simulink library "pixhawk_slib_adv"  (R2017b)
settings: Solver=ode45  StartTime=0.0  StopTime=10.0  RelTol=1e-3
undefined symbols (not defined in the file or in its folder): Earth, earthRadius, ModelInit_AngEuler, ModelInit_PosE, ModelInit_RateB, ModelInit_RPM, ModelInit_VelB, ModelParam_envAltitude, ModelParam_GPSLatLong, ModelParam_motorCr, ModelParam_motorJm, ModelParam_motorT, ModelParam_motorWb, ModelParam_noisePowerIMU, ModelParam_rotorCm, ModelParam_rotorCt, ModelParam_uavCCm, ModelParam_uavCd, ModelParam_uavDearo, ModelParam_uavJ, ModelParam_uavMass, ModelParam_uavR, ModelParam_uavType, Receive, Send, WGS84
libraries: etargetslib x11, dspnetwork x9, simulink x8, sharedtransform x5, aerolibtransform2 x4, aerolibutil x4, pixhawk_slib_adv x3, aerolibfltsims x3, shared6dof x1, aerolibobsolete x1, aerolibasang x1, aerolibatmos2 x1
(part 2 of 3)

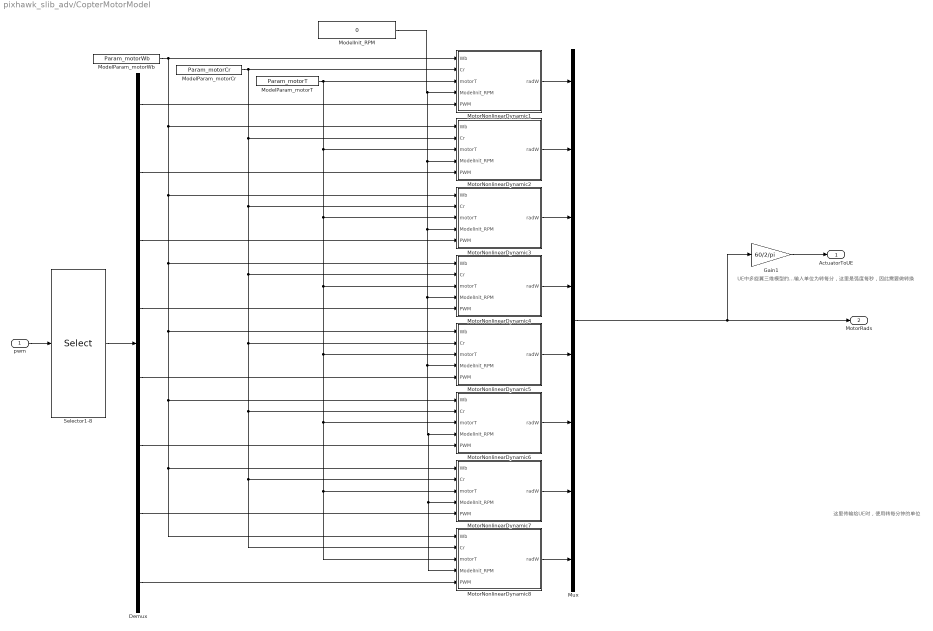
== system pixhawk_slib_adv/CopterMotorModel ==
  note: UE中多旋翼三维模型的输入单位为转每分，这里是弧度每秒，因此需要做转换
  note: 这里传输给UE时，使用转每分钟的单位
  pwm : Inport
  Demux : Demux  Outputs=8
  Gain1 : Gain  Gain=60/2/pi
  ModelInit_RPM : Constant  Value=0
  ModelParam_motorCr : Constant  Value=Param_motorCr
  ModelParam_motorT : Constant  Value=Param_motorT
  ModelParam_motorWb : Constant  Value=Param_motorWb
  MotorNonlinearDynamic1 : Subsystem  TreatAsAtomicUnit=on
  MotorNonlinearDynamic2 : Subsystem  TreatAsAtomicUnit=on
  MotorNonlinearDynamic3 : Subsystem  TreatAsAtomicUnit=on
  MotorNonlinearDynamic4 : Subsystem  TreatAsAtomicUnit=on
  MotorNonlinearDynamic5 : Subsystem  TreatAsAtomicUnit=on
  MotorNonlinearDynamic6 : Subsystem  TreatAsAtomicUnit=on
  MotorNonlinearDynamic7 : Subsystem  TreatAsAtomicUnit=on
  MotorNonlinearDynamic8 : Subsystem  TreatAsAtomicUnit=on
  Mux : Mux  Inputs=8
  Selector1-8 : Selector  InputPortWidth=16  IndexOptions=Index vector (dialog)  Indices=[1:8]  OutputSizes=1
  ActuatorToUE : Outport
  MotorRads : Outport  Port=2
  wires:
  Mux/1 -> Gain1/1, MotorRads/1
  Demux/1 -> MotorNonlinearDynamic1/5(PWM)
  MotorNonlinearDynamic1/1(radW) -> Mux/1
  ModelParam_motorCr/1 -> MotorNonlinearDynamic1/2(Cr), MotorNonlinearDynamic2/2(Cr), MotorNonlinearDynamic3/2(Cr), MotorNonlinearDynamic4/2(Cr), MotorNonlinearDynamic5/2(Cr), MotorNonlinearDynamic6/2(Cr), MotorNonlinearDynamic8/2(Cr), MotorNonlinearDynamic7/2(Cr)
  ModelParam_motorWb/1 -> MotorNonlinearDynamic1/1(Wb), MotorNonlinearDynamic2/1(Wb), MotorNonlinearDynamic3/1(Wb), MotorNonlinearDynamic4/1(Wb), MotorNonlinearDynamic5/1(Wb), MotorNonlinearDynamic6/1(Wb), MotorNonlinearDynamic8/1(Wb), MotorNonlinearDynamic7/1(Wb)
  Demux/2 -> MotorNonlinearDynamic2/5(PWM)
  Demux/3 -> MotorNonlinearDynamic3/5(PWM)
  Demux/4 -> MotorNonlinearDynamic4/5(PWM)
  Demux/5 -> MotorNonlinearDynamic5/5(PWM)
  Demux/6 -> MotorNonlinearDynamic6/5(PWM)
  Demux/7 -> MotorNonlinearDynamic7/5(PWM)
  Demux/8 -> MotorNonlinearDynamic8/5(PWM)
  ModelParam_motorT/1 -> MotorNonlinearDynamic2/3(motorT), MotorNonlinearDynamic3/3(motorT), MotorNonlinearDynamic4/3(motorT), MotorNonlinearDynamic5/3(motorT), MotorNonlinearDynamic6/3(motorT), MotorNonlinearDynamic8/3(motorT), MotorNonlinearDynamic7/3(motorT), MotorNonlinearDynamic1/3(motorT)
  MotorNonlinearDynamic2/1(radW) -> Mux/2
  MotorNonlinearDynamic8/1(radW) -> Mux/8
  MotorNonlinearDynamic7/1(radW) -> Mux/7
  MotorNonlinearDynamic6/1(radW) -> Mux/6
  MotorNonlinearDynamic5/1(radW) -> Mux/5
  MotorNonlinearDynamic4/1(radW) -> Mux/4
  MotorNonlinearDynamic3/1(radW) -> Mux/3
  Selector1-8/1 -> Demux/1
  ModelInit_RPM/1 -> MotorNonlinearDynamic8/4(ModelInit_RPM), MotorNonlinearDynamic7/4(ModelInit_RPM), MotorNonlinearDynamic6/4(ModelInit_RPM), MotorNonlinearDynamic5/4(ModelInit_RPM), MotorNonlinearDynamic4/4(ModelInit_RPM), MotorNonlinearDynamic3/4(ModelInit_RPM), MotorNonlinearDynamic2/4(ModelInit_RPM), MotorNonlinearDynamic1/4(ModelInit_RPM)
  Gain1/1 -> ActuatorToUE/1
  pwm/1 -> Selector1-8/1

== system pixhawk_slib_adv/GroundModel ==
  tz : Inport
  6DOF : Inport  Port=2
  Bus Creator : BusCreator  Inputs=2
  Constant : Constant  Value=ModelChoice
  Multiport Switch : MultiPortSwitch  Inputs=2  DataPortIndices=1
  Subsystem1 : Subsystem
  "Subsystem2 " : Subsystem
  fm : Outport
  wires:
  tz/1 -> Bus Creator/1
  6DOF/1 -> Bus Creator/2
  Multiport Switch/1 -> fm/1
  Constant/1 -> Multiport Switch/1
  Subsystem1/1(Out1) -> Multiport Switch/2
  "Subsystem2 "/1(Out1) -> Multiport Switch/3
  Bus Creator/1 -> "Subsystem2 "/1(In1), Subsystem1/1(In1)

== system pixhawk_slib_adv/PX4FaultInParamsSend ==
  note: struct PX4ModelInParams {
      | int checksum ; //1234567891
      | int Bitmask ;
      | double InParams [ 32 ];
      | };
  note: This message will be sent to PX4 DLL model's Params signals ModelInParams [32].
      | The checksum should be set to 1234567891, and the data should be sent to port 30100+(i-1)*2.
      | The bitmask specify which dimension of 32-D ModelInParams vector.
  Bitmask : Inport  OutDataTypeStr=int32  PortDimensions=1
  InParams : Inport  Port=2  OutDataTypeStr=single  PortDimensions=32
  Data Type Conversion1 : DataTypeConversion  OutDataTypeStr=int32
  Data Type Conversion2 : DataTypeConversion  OutDataTypeStr=double
  Data Type Conversion3 : DataTypeConversion  OutDataTypeStr=int32
  PayLoad : etargetslib/Byte Pack  datatypes={'int32','int32','double'}  byteAlign=4
  UDP Send : dspnetwork/UDP Send  remoteURL=TargetIP  remotePort=30100 + CopterID*2 -2  localURL='0.0.0.0'  localPortSource=Automatically determine  localPort=-1  sampletime=-1  blockPlatform=[]  separateLengthPort=0
      settings: SourceProductName=DSP System Toolbox  SourceProductBaseCode=DS
  checksum : Constant  Value=1234567891  OutDataTypeStr=Inherit: Inherit via back propagation
  wires:
  InParams/1 -> Data Type Conversion2/1
  Bitmask/1 -> Data Type Conversion1/1
  PayLoad/1 -> UDP Send/1
  Data Type Conversion1/1 -> PayLoad/2
  Data Type Conversion2/1 -> PayLoad/3
  checksum/1 -> Data Type Conversion3/1
  Data Type Conversion3/1 -> PayLoad/1

== system pixhawk_slib_adv/PX4SILIntFloatSend ==
  note: struct PX4SILIntFloat {
      | int checksum ;
      | int CopterID ;
      | int inSILInts [ 8 ];
      | float inSILFLoats [ 20 ];
      | }
  note: This message will be sent to PX4 DLL model's input signals inSILInts[8] and inSILFloats[20].
      | The checksum should be set to 1234567897, and the data should be sent to port 30100+(i-1)*2
  inSILInts : Inport  OutDataTypeStr=int32  PortDimensions=8
  inSILFloats : Inport  Port=2  OutDataTypeStr=single  PortDimensions=20
  CopterID : Constant  OutDataTypeStr=Inherit: Inherit via back propagation
  Data Type Conversion1 : DataTypeConversion  OutDataTypeStr=int32
  Data Type Conversion2 : DataTypeConversion  OutDataTypeStr=single
  Data Type Conversion3 : DataTypeConversion  OutDataTypeStr=int32
  Mux : Mux  Inputs=2
  PayLoad : etargetslib/Byte Pack  datatypes={'int32','int32','single'}  byteAlign=8
  UDP Send : dspnetwork/UDP Send  remoteURL=TargetIP  remotePort=30100 + CopterID*2 -2  localURL='0.0.0.0'  localPortSource=Automatically determine  localPort=-1  sampletime=-1  blockPlatform=[]  separateLengthPort=0
      settings: SourceProductName=DSP System Toolbox  SourceProductBaseCode=DS
  checksum : Constant  Value=1234567897  OutDataTypeStr=Inherit: Inherit via back propagation
  wires:
  inSILFloats/1 -> Data Type Conversion2/1
  inSILInts/1 -> Data Type Conversion1/1
  PayLoad/1 -> UDP Send/1
  Data Type Conversion1/1 -> PayLoad/2
  Data Type Conversion2/1 -> PayLoad/3
  checksum/1 -> Mux/1
  Mux/1 -> Data Type Conversion3/1
  Data Type Conversion3/1 -> PayLoad/1
  CopterID/1 -> Mux/2

== system pixhawk_slib_adv/PlaneGroundModel ==
  note: GroundSupportModel
  note: From Earth to body frame
  note: 计算重量
  "tZ " : Inport
  6DOF : Inport  Port=2
  Bus Selector : BusSelector  OutputSignals=Xe,Ve,Eular(rad),DCM,wb,mass,gravity
  Direction Cosine Matrix to Quaternions : sharedtransform/Direction Cosine Matrix  to Quaternions
      settings: SourceProductName=Aerospace Blockset  SourceProductBaseCode=AE
  Direction Cosine Matrix to Quaternions1 : sharedtransform/Direction Cosine Matrix  to Quaternions
      settings: SourceProductName=Aerospace Blockset  SourceProductBaseCode=AE
  Euler to DCM : aerolibtransform2/Wind Angles to  Direction Cosine Matrix
      settings: SourceProductName=Aerospace Blockset  SourceProductBaseCode=AE
  Ground Model : MATLAB Function  TreatAsAtomicUnit=on
  Mux : Mux  Inputs=2
  OnGroundFaceup : Subsystem
  Product : Product  Multiplication=Matrix(*)
  Product1 : Product
  Quaternion Inverse : aerolibutil/Quaternion Inverse
      settings: SourceProductName=Aerospace Blockset
  Quaternion Multiplication : aerolibutil/Quaternion Multiplication
  FM : Outport
  wires:
  "tZ "/1 -> Ground Model/6(terrainZ)
  Ground Model/2(M1) -> Mux/2  "Mb"
  Product/1 -> Mux/1  "Fb"
  Quaternion Multiplication/1 -> Ground Model/5(Quet)
  Quaternion Inverse/1 -> Quaternion Multiplication/1
  Direction Cosine Matrix to Quaternions1/1 -> Quaternion Inverse/1
  Euler to DCM/1 -> Direction Cosine Matrix to Quaternions1/1
  Direction Cosine Matrix to Quaternions/1 -> Quaternion Multiplication/2
  Ground Model/1(F1) -> Product/2
  Bus Selector/4 -> Direction Cosine Matrix to Quaternions/1, Product/1  "<DCM>"
  Bus Selector/5 -> Ground Model/2(wb)  "<wb>"
  6DOF/1 -> Bus Selector/1
  Bus Selector/2 -> Ground Model/4(Ve)  "<Ve>"
  Bus Selector/1 -> Ground Model/3(Xe)  "<Xe>"
  Bus Selector/3 -> OnGroundFaceup/1(Eular(rad))  "<Eular(rad)>"
  OnGroundFaceup/1(y) -> Euler to DCM/1
  Product1/1 -> Ground Model/1(mg)  "mg"
  Bus Selector/6 -> Product1/1  "<mass>"
  Bus Selector/7 -> Product1/2  "<gravity>"
  Mux/1 -> FM/1

== system pixhawk_slib_adv/RflyChangeMap ==
  MapNameorID : Inport
  Data Type Conversion8 : DataTypeConversion  OutDataTypeStr=int32
  Data Type Conversion9 : DataTypeConversion  OutDataTypeStr=uint8
  MATLAB Function : MATLAB Function  TreatAsAtomicUnit=on
  PayLoad1 : etargetslib/Byte Pack  datatypes={'int32','uint8'}  byteAlign=4
  UDP Send1 : dspnetwork/UDP Send  remoteURL='127.0.0.1'  remotePort=20010  localURL='0.0.0.0'  localPortSource=Automatically determine  localPort=-1  sampletime=-1  blockPlatform=[]  separateLengthPort=0
      settings: SourceProductName=DSP System Toolbox  SourceProductBaseCode=DS
  checkSum : Constant  Value=1234567890
  wires:
  MapNameorID/1 -> MATLAB Function/1(input)
  checkSum/1 -> Data Type Conversion8/1
  Data Type Conversion9/1 -> PayLoad1/2
  PayLoad1/1 -> UDP Send1/1
  Data Type Conversion8/1 -> PayLoad1/1
  MATLAB Function/1(data) -> Data Type Conversion9/1

== system pixhawk_slib_adv/SensorOutput ==
  note: Struct MavHILStateQuat{
      | uint64_t time_usec; /*< Timestamp (microseconds since UNIX epoch or microseconds since system boot)*/
      | float attitude_quaternion [ 4 ]; /*< Vehicle attitude expressed as normalized quaternion in w, x, y, z order (with 1 0 0 0 being the null-rotation)*/
      | float rollspeed; /*< Body frame roll / phi angular speed (rad/s)*/
      | float pitchspeed; /*< Body frame pitch / theta angular speed (rad/s)*/
      | float yawspeed; /*< Body frame yaw / psi angular speed (rad/s)*/
      | int32_t lat; /*< Latitude, expressed as * 1E7*/
      | int32_t lon; /*< Longitude, expressed as * 1E7*/
      | int32_t alt; /*< Altitude in meters, expressed as * 1000 (millimeters)*/
      | int16_t vx; /*< Ground X Speed (Latitude), expressed as cm/s*/
      | int16_t vy; /*< Ground Y Speed (Longitude), expressed as cm/s*/
      | int16_t vz; /*< Ground Z Speed (Altitude), expressed as cm/s*/
      | uint16_t ind_airspeed; /*< Indicated airspeed, expressed as cm/s*/
      | uint16_t true_airspeed; /*< True airspeed, expressed as cm/s*/
      | int16_t xacc; /*< X acceleration (mg)*/
      | int16_t yacc; /*< Y acceleration (mg)*/
      | int16_t zacc; /*< Z acceleration (mg)*/
      | };
  6DOF : Inport
  Bus Selector : BusSelector  OutputSignals=Ve,DCM,wb,dwb/dt,AccB,WindB,PosGPS,gravity
  Clock1 : Clock
  Gain_clock : Gain  Gain=1E6
  HILGPSModel : Subsystem
  HILSensorMavModel : Subsystem
  HILSensor30d : Outport
  HILGPS30d : Outport  Port=2
  wires:
  Bus Selector/8 -> HILSensorMavModel/2(Gravity)  "<gravity>"
  Bus Selector/2 -> HILSensorMavModel/7(DCMbe)  "<DCM>"
  Bus Selector/4 -> HILSensorMavModel/5(dwt)  "<dwb/dt>"
  Bus Selector/7 -> HILSensorMavModel/3(GPSPos), HILGPSModel/3(PosGPS)  "<PosGPS>"
  Bus Selector/5 -> HILSensorMavModel/6(Ab)  "<AccB>"
  Bus Selector/1 -> HILGPSModel/2(Ve)  "<Ve>"
  Bus Selector/3 -> HILSensorMavModel/4(wb)  "<wb>"
  6DOF/1 -> Bus Selector/1
  Clock1/1 -> Gain_clock/1
  Gain_clock/1 -> HILSensorMavModel/1(time_usec), HILGPSModel/1(time_usec)  "time_usec"
  Bus Selector/6 -> HILSensorMavModel/8(windB)  "<WindB>"
  HILSensorMavModel/1(HILSensor30d) -> HILSensor30d/1
  HILGPSModel/1(HILGPS30d) -> HILGPS30d/1

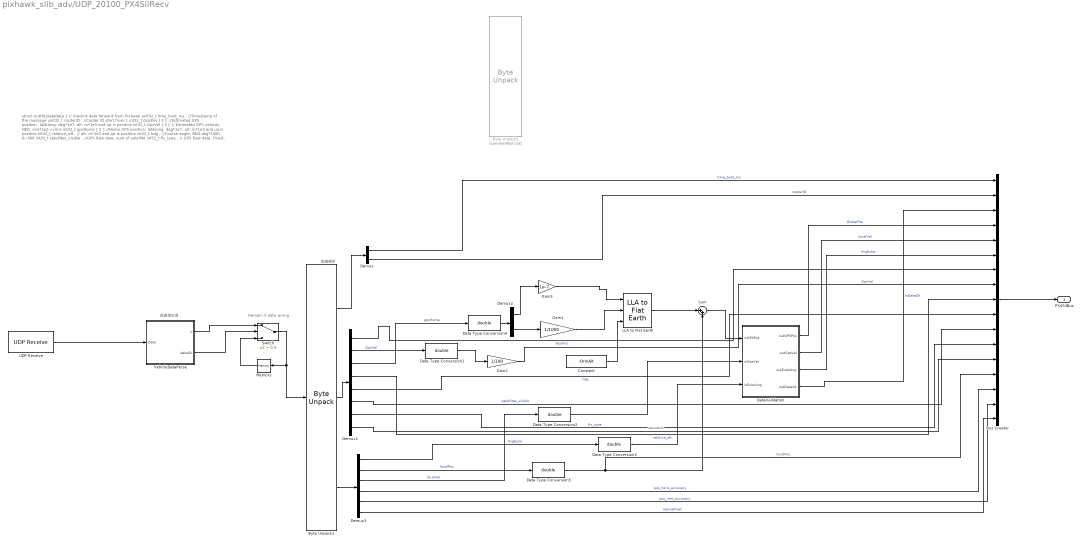
== system pixhawk_slib_adv/UDP_20100_PX4SilRecv ==
  note: 数据解析
  note: 数据预处理
  note: Remain if data wrong
  note: struct outHILStateData { // mavlink data forward from Pixhawk
      | uint32_t time_boot_ms ; //Timestamp of the message
      | uint32_t copterID ; //Copter ID start from 1
      | int32_t GpsPos [ 3 ]; //Estimated GPS position，lat&long: deg*1e7, alt: m*1e3 and up is positive
      | int32_t GpsVel [ 3 ]; // Estimated GPS velocity, NED, m/s*1e2->cm/s
      | int32_t gpsHome [ 3 ]; //Home GPS position, lat&long: deg*1e7, alt: m*1e3 and up is positive
      | int32_t relative_alt ; // alt: m*1e3 and up is positive
      | int32_t hdg ; //Course angle, NED,deg*1000, 0~360
      | int32_t satellites_visible ; //GPS Raw data, sum of satellite
      | int32_t fix_type ; // GPS Raw data, Fixed type, 3 for fixed (good precision)
      | int32_t resrveInit ; //Int, reserve for the future use
      | float AngEular [ 3 ]; //Estimated Euler angle, unit: rad/s
      | float localPos [ 3 ]; //Estimated locoal position, NED, unit: m
      | float localVel [ 3 ]; // Estimated locoal velocity, NED, unit: m/s
      | float pos_horiz_accuracy ; // GPS horizontal accuracy, unit: m
      | float pos_vert_accuracy ; // GPS vertical accuracy, unit: m
      | float resrveFloat ; //float, reserve for the future use
      | }
  Bus Creator : BusCreator  Inputs=17
  Byte Unpack1 : etargetslib/Byte Unpack  dimensions={2,14,12}  datatypes={'uint32','int32','single'}  byteAlign=8
  Byte Unpack2 : etargetslib/Byte Unpack  Commented=on  dimensions={1,1,1,3,3,3,4,8,3,3,3}  datatypes={'int32','int32','double','single','single','single','single','single','single','single','double'}  byteAlign=1
  Constant : Constant  Value=-OrinAlt
  Data Type Conversion{1..5} (5 alike) : DataTypeConversion  OutDataTypeStr=double
  DataValidation : MATLAB Function  TreatAsAtomicUnit=on
  Demux : Demux  Outputs=2
  Demux1 : Demux  Outputs=[3,3,3,1,1,1,1,1]
  Demux2 : Demux  Outputs=[2,1]
  Demux3 : Demux  Outputs=[3,3,3,1,1,1]
  Gain1 : Gain  Gain=1/1000
  Gain2 : Gain  Gain=1/100
  Gain5 : Gain  Gain=1e-7
  LLA to Flat Earth : aerolibtransform2/LLA to Flat Earth  units=Metric (MKS)  ptype=Earth (WGS84)  F=1/298.257223563  R=6378137  LL0=OrinLatLon  psi=0
      settings: SourceProductName=Aerospace Blockset  SourceProductBaseCode=AE
  Memory : Memory  InitialCondition=uint8(zeros(112,1))
  Sum : Sum  Inputs=|++
  Switch : Switch  Criteria=u2 > Threshold  Threshold=0.5
  UDP Receive : dspnetwork/UDP Receive  localURL='0.0.0.0'  localPort=20100 + CopterID*2 -1  remoteURL='0.0.0.0'  remotePort=-1  recvBufferSize=8192  dims=255  signalDatatype=uint8  isVarSize=on  showBlockingTime=off  blockingTime=0  sampletime=-1  blockPlatform=[]
      settings: SourceProductName=DSP System Toolbox  SourceProductBaseCode=DS
  VehicleDataPerse : MATLAB Function  TreatAsAtomicUnit=on
  PX4SilBus : Outport
  wires:
  VehicleDataPerse/2(dataOk) -> Switch/2
  UDP Receive/1 -> VehicleDataPerse/1(Data)
  VehicleDataPerse/1(y) -> Switch/1
  Switch/1 -> Memory/1, Byte Unpack1/1
  Memory/1 -> Switch/3
  Byte Unpack1/1 -> Demux/1
  Demux/1 -> Bus Creator/1  "time_boot_ms"
  Demux/2 -> Bus Creator/2  "copterID"
  Byte Unpack1/2 -> Demux1/1
  Demux1/2 -> Data Type Conversion1/1  "GpsVel"
  Demux2/1 -> Gain5/1
  Demux2/2 -> Gain1/1
  Gain1/1 -> LLA to Flat Earth/2
  Demux1/1 -> Bus Creator/7  "GpsPos"
  LLA to Flat Earth/1 -> Sum/1
  Data Type Conversion1/1 -> Gain2/1
  Data Type Conversion3/1 -> DataValidation/3(inEulerAng)
  Gain5/1 -> LLA to Flat Earth/1
  Data Type Conversion4/1 -> Demux2/1
  Byte Unpack1/3 -> Demux3/1
  Demux1/3 -> Data Type Conversion4/1  "gpsHome"
  Demux1/4 -> Bus Creator/9  "relative_alt"
  Demux1/5 -> Bus Creator/10  "hdg"
  Demux1/6 -> Bus Creator/11  "satellites_visible"
  Demux1/7 -> Bus Creator/12  "fix_type"
  Demux3/1 -> Data Type Conversion3/1  "AngEular"
  Demux3/2 -> Data Type Conversion5/1  "localPos"
  Demux3/3 -> Data Type Conversion2/1  "localVel"
  Demux3/4 -> Bus Creator/15  "pos_horiz_accuracy"
  Demux3/5 -> Bus Creator/16  "pos_vert_accuracy"
  Demux1/8 -> Bus Creator/13  "resrveInit"
  Demux3/6 -> Bus Creator/17  "resrveFloat"
  Constant/1 -> LLA to Flat Earth/3
  DataValidation/1(outGPSPos) -> Bus Creator/4  "GlobalPos"
  DataValidation/2(outGpsVel) -> Bus Creator/5  "localVel"
  DataValidation/3(outEulerAng) -> Bus Creator/6  "AngEular"
  DataValidation/4(outDataOk) -> Bus Creator/3  "IsDataOK"
  Data Type Conversion2/1 -> DataValidation/2(inGpsVel)
  Gain2/1 -> Bus Creator/8  "GpsVel"
  Data Type Conversion5/1 -> Bus Creator/14, Sum/2  "localPos"
  Sum/1 -> DataValidation/1(inGPSPos)
  Bus Creator/1 -> PX4SilBus/1

== system pixhawk_slib_adv/UDP_30100_TrueSimRecv ==
  note: % //FULL完整模式，输出到RflySim3D的数据
      | % struct SOut2Simulator {
      | %     int checksum; // 校验码123456789，必须设定为本值，才会认为是有效数据
      | %     int copterID;  //飞机ID序号
      | %     int vehicleType;  //载具样式ID，对应UE的XML中ClassID
      | %     int reserv; //备用标志位，Int型，将来用于表示碰撞、或大地图等标识
      | %     float VelE[3];   //速度，北东地，单位米/s
      | %     float AngEuler[3];  //欧拉角，滚转俯仰偏航，单位弧度
      | %     float AngQuatern[4]; //姿态四元数向量，w x y z
      | %     float MotorRPMS[8];  //执行器偏转量或转速，旋翼类对应RPM转每分
      | %     float AccB[3];       //载具机体FRD坐标系下加速度
      | %     float RateB[3];      //载具机体FRD坐标系下角速度，pqr，单位rad/s
      | %     double runnedTime; //时间戳，仿真开始为0时刻。
      | %     double PosE[3];   //北东地位置，单位米，z向下为正
      | %     double PosGPS[3];    //载具纬度、经度、高度向量，单位度和米，高度向上为正
      | % };
      | % // Python解码标识4i24f7d，数据长度168字节
  note: 数据解析
  Bus Creator : BusCreator  Inputs=13
  Demux2 : Demux  Outputs=35
  Mux{,1,4..7} (6 alike) : Mux  Inputs=3
  Mux2 : Mux
  Mux3 : Mux  Inputs=8
  Terminator : Terminator
  UDP Receive : dspnetwork/UDP Receive  localURL='0.0.0.0'  localPort=30100 + CopterID * 2 -1  remoteURL='0.0.0.0'  remotePort=-1  recvBufferSize=8192  dims=255  signalDatatype=uint8  isVarSize=on  showBlockingTime=off  blockingTime=0  sampletime=-1  blockPlatform=[]
      settings: SourceProductName=DSP System Toolbox  SourceProductBaseCode=DS
  VehicleDataPerse1 : MATLAB Function  TreatAsAtomicUnit=on
  SimData : Outport
  wires:
  UDP Receive/1 -> VehicleDataPerse1/1(Data)
  VehicleDataPerse1/1(y) -> Demux2/1
  Demux2/2 -> Bus Creator/1  "copterID"
  Demux2/3 -> Bus Creator/2  "vehicleType"
  Demux2/4 -> Bus Creator/3  "reserv"
  Demux2/5 -> Mux/1
  Demux2/6 -> Mux/2
  Demux2/7 -> Mux/3
  Mux/1 -> Bus Creator/4  "VelE"
  Demux2/8 -> Mux1/1
  Demux2/9 -> Mux1/2
  Demux2/10 -> Mux1/3
  Mux1/1 -> Bus Creator/5  "AngEuler"
  Demux2/11 -> Mux2/1
  Demux2/12 -> Mux2/2
  Demux2/13 -> Mux2/3
  Demux2/14 -> Mux2/4
  Mux2/1 -> Bus Creator/6  "AngQuatern"
  Demux2/15 -> Mux3/1
  Demux2/16 -> Mux3/2
  Demux2/17 -> Mux3/3
  Demux2/18 -> Mux3/4
  Demux2/19 -> Mux3/5
  Demux2/20 -> Mux3/6
  Demux2/21 -> Mux3/7
  Demux2/22 -> Mux3/8
  Mux3/1 -> Bus Creator/7  "MotorRPMS"
  Demux2/23 -> Mux4/1
  Demux2/24 -> Mux4/2
  Demux2/25 -> Mux4/3
  Mux4/1 -> Bus Creator/8  "AccB"
  Demux2/26 -> Mux5/1
  Demux2/27 -> Mux5/2
  Demux2/28 -> Mux5/3
  Mux5/1 -> Bus Creator/9  "RateB"
  Demux2/29 -> Bus Creator/10  "runnedTime"
  Demux2/30 -> Mux6/1
  Demux2/31 -> Mux6/2
  Demux2/32 -> Mux6/3
  Mux6/1 -> Bus Creator/11  "PosE"
  Demux2/33 -> Mux7/1
  Demux2/34 -> Mux7/2
  Demux2/35 -> Mux7/3
  Mux7/1 -> Bus Creator/12  "PosGPS"
  Bus Creator/1 -> SimData/1
  Demux2/1 -> Terminator/1
  VehicleDataPerse1/2(dataOk) -> Bus Creator/13  "IsDataOK"

== system pixhawk_slib_adv/UDP_40100_RflyPx4Recv ==
  note: struct PX4ExtMsg {
      | int checksum ; //1234567898
      | int CopterID ;
      | double runnedTime ; //Current stamp (s)
      | float controls [ 8 ];
      | }
  note: 数据解析
  note: 数据预处理
  note: 如果数据不正确则用前一时刻数据
  Byte Unpack1 : etargetslib/Byte Unpack  dimensions={2,1,8}  datatypes={'int32','double','single'}  byteAlign=8
  CopterID : Display
  Demux : Demux  Outputs=2
  Memory : Memory  InitialCondition=uint8(zeros(48,1))
  Switch : Switch  Criteria=u2 > Threshold  Threshold=0.5
  UDP Receive : dspnetwork/UDP Receive  localURL='0.0.0.0'  localPort=40100 + CopterID * 2 -1  remoteURL='0.0.0.0'  remotePort=-1  recvBufferSize=8192  dims=120  signalDatatype=uint8  isVarSize=on  showBlockingTime=off  blockingTime=0  sampletime=-1  blockPlatform=[]
      settings: SourceProductName=DSP System Toolbox  SourceProductBaseCode=DS
  VehicleDataPerse : MATLAB Function  TreatAsAtomicUnit=on
  checksum : Display
  runnedTime : Display
  controls : Outport
  wires:
  VehicleDataPerse/2(dataOk) -> Switch/2
  UDP Receive/1 -> VehicleDataPerse/1(Data)
  VehicleDataPerse/1(y) -> Switch/1
  Switch/1 -> Memory/1, Byte Unpack1/1
  Memory/1 -> Switch/3
  Byte Unpack1/1 -> Demux/1
  Demux/1 -> checksum/1
  Demux/2 -> CopterID/1
  Byte Unpack1/2 -> runnedTime/1
  Byte Unpack1/3 -> controls/1

== system pixhawk_slib_adv/sendUE4ExtAct ==
  CopterID : Inport
  "ActExt  " : Inport  Port=2
  UDP Send2 : dspnetwork/UDP Send  remoteURL='127.0.0.1'  remotePort=20010  localURL='0.0.0.0'  localPortSource=Automatically determine  localPort=-1  sampletime=-1  blockPlatform=[]  separateLengthPort=0
      settings: SourceProductName=DSP System Toolbox  SourceProductBaseCode=DS
  Ue4ExtMsgEncoder : Subsystem
  wires:
  CopterID/1 -> Ue4ExtMsgEncoder/1(copterID)
  "ActExt  "/1 -> Ue4ExtMsgEncoder/2(pwm)
  Ue4ExtMsgEncoder/1(Ue4ExtMsg) -> UDP Send2/1

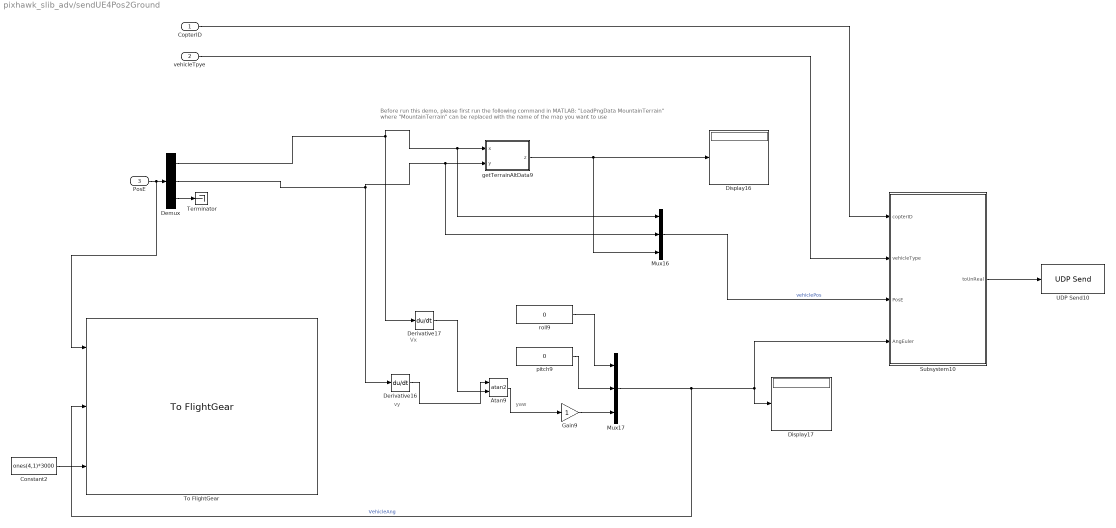
== system pixhawk_slib_adv/sendUE4Pos2Ground ==
  note: vy
  note: Vx
  note: Before run this demo, please first run the following command in MATLAB: "LoadPngData MountainTerrain"
      | where "MountainTerrain" can be replaced with the name of the map you want to use
  note: yaw
  CopterID : Inport
  vehicleTpye : Inport  Port=2
  PosE : Inport  Port=3
  Atan9 : Trigonometry  Operator=atan2
  Constant2 : Constant  Value=ones(4,1)*3000
  Demux : Demux  Outputs=3
  Derivative16 : Derivative
  Derivative17 : Derivative
  Display16 : Display
  Display17 : Display
  Gain9 : Gain
  Mux16 : Mux  Inputs=3
  Mux17 : Mux  Inputs=3
  Subsystem10 : Subsystem
  Terminator : Terminator
  To FlightGear : pixhawk_slib_adv/sendUE4PosFull/To FlightGear  SystemSampleTime=-1  Latency=0  AutoFrameSizeCalculation=off
      settings: SourceProductName=Pixhawk Target Blocks
  UDP Send10 : dspnetwork/UDP Send  remoteURL='127.0.0.1'  remotePort=20010  localURL='0.0.0.0'  localPortSource=Automatically determine  localPort=-1  sampletime=-1  blockPlatform=[]  separateLengthPort=0
      settings: SourceProductName=DSP System Toolbox  SourceProductBaseCode=DS
  getTerrainAltData9 : MATLAB Function  TreatAsAtomicUnit=on
  pitch9 : Constant  Value=0
  roll9 : Constant  Value=0
  wires:
  pitch9/1 -> Mux17/2
  Gain9/1 -> Mux17/3
  Mux17/1 -> To FlightGear/2, Display17/1, Subsystem10/4(AngEuler)  "VehicleAng"
  Derivative17/1 -> Atan9/2
  Demux/2 -> Derivative16/1, Mux16/2, getTerrainAltData9/2(y)
  vehicleTpye/1 -> Subsystem10/2(vehicleType)
  CopterID/1 -> Subsystem10/1(copterID)
  Subsystem10/1(toUnReal) -> UDP Send10/1
  Atan9/1 -> Gain9/1
  roll9/1 -> Mux17/1
  Demux/1 -> Mux16/1, getTerrainAltData9/1(x), Derivative17/1
  Derivative16/1 -> Atan9/1
  Mux16/1 -> Subsystem10/3(PosE)  "vehiclePos"
  getTerrainAltData9/1(z) -> Mux16/3, Display16/1
  PosE/1 -> To FlightGear/1, Demux/1
  Demux/3 -> Terminator/1
  Constant2/1 -> To FlightGear/3

== system pixhawk_slib_adv/sendUE4PosFull ==
  copterID : Inport  PortDimensions=1
  vehicleType : Inport  Port=2  PortDimensions=1
  MotorRPMS : Inport  Port=3
  VelE : Inport  Port=4
  PosE : Inport  Port=5  PortDimensions=3
  RateB : Inport  Port=6
  AngEuler : Inport  Port=7  PortDimensions=3
  Clock : Clock
  Constant1 : Constant  Value=[0,0,0,0]
  Constant3 : Constant  Value=[0,0,0]
  Constant5 : Constant  Value=[0,0,0]
  Subsystem : Subsystem
  To FlightGear : Subsystem
      mask Display: image('./icon/FlightGear.png');
  UDP Send : dspnetwork/UDP Send  remoteURL='127.0.0.1'  remotePort=20010  localURL='0.0.0.0'  localPortSource=Automatically determine  localPort=-1  sampletime=-1  blockPlatform=[]  separateLengthPort=0
      settings: SourceProductName=DSP System Toolbox  SourceProductBaseCode=DS
  wires:
  RateB/1 -> Subsystem/10(RateB)
  Constant5/1 -> Subsystem/11(PosGPS)
  Constant3/1 -> Subsystem/9(AccB)
  Subsystem/1(toUnReal) -> UDP Send/1
  VelE/1 -> Subsystem/4("VelE ")
  Clock/1 -> Subsystem/3(runnedTime)
  MotorRPMS/1 -> To FlightGear/3(MotorPWMs), Subsystem/8(MotorRPMS)
  Constant1/1 -> Subsystem/7(AngQuatern)
  AngEuler/1 -> To FlightGear/2(AngEuler), Subsystem/6(AngEuler)
  PosE/1 -> To FlightGear/1(PosE), Subsystem/5(PosE)
  copterID/1 -> Subsystem/1(copterID)
  vehicleType/1 -> Subsystem/2(vehicleType)

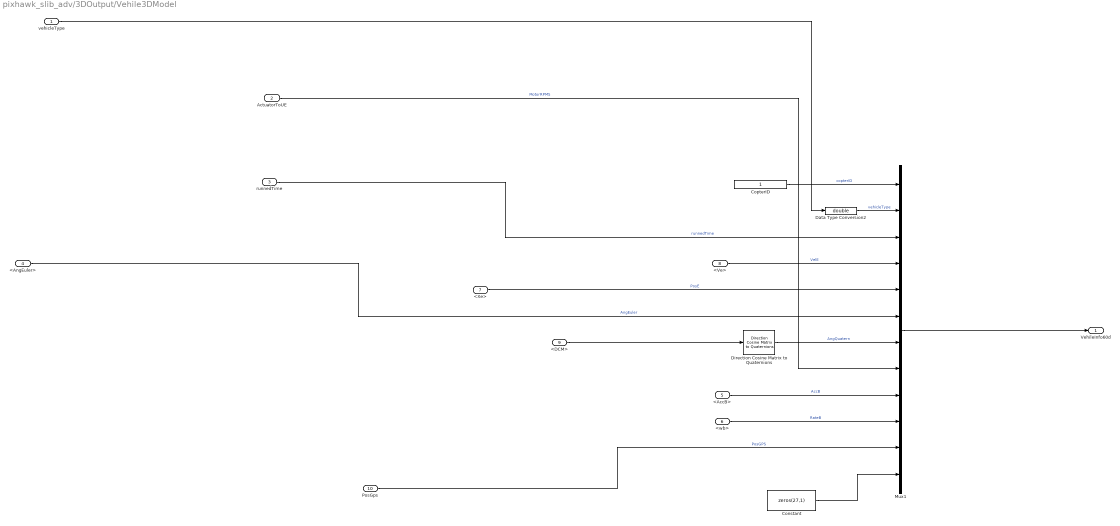
== system pixhawk_slib_adv/3DOutput/Vehile3DModel ==
  vehicleType : Inport
  ActuatorToUE : Inport  Port=2
  runnedTime : Inport  Port=3
  <AngEuler> : Inport  Port=4
  <AccB> : Inport  Port=5
  <wb> : Inport  Port=6
  <Xe> : Inport  Port=7
  <Ve> : Inport  Port=8
  <DCM> : Inport  Port=9
  PosGps : Inport  Port=10
  Constant : Constant  Value=zeros(27,1)
  CopterID : Constant
  Data Type Conversion2 : DataTypeConversion  OutDataTypeStr=double
  Direction Cosine Matrix to Quaternions : sharedtransform/Direction Cosine Matrix  to Quaternions
      settings: SourceProductName=Aerospace Blockset  SourceProductBaseCode=AE
  Mux1 : Mux  Inputs=12
  VehileInfo60d : Outport
  wires:
  Mux1/1 -> VehileInfo60d/1
  Data Type Conversion2/1 -> Mux1/2  "vehicleType"
  runnedTime/1 -> Mux1/3  "runnedTime"
  <AccB>/1 -> Mux1/9  "AccB"
  CopterID/1 -> Mux1/1  "copterID"
  Direction Cosine Matrix to Quaternions/1 -> Mux1/7  "AngQuatern"
  <wb>/1 -> Mux1/10  "RateB"
  <AngEuler>/1 -> Mux1/6  "AngEuler"
  <Xe>/1 -> Mux1/5  "PosE"
  vehicleType/1 -> Data Type Conversion2/1
  <Ve>/1 -> Mux1/4  "VelE"
  ActuatorToUE/1 -> Mux1/8  "MotorRPMS"
  <DCM>/1 -> Direction Cosine Matrix to Quaternions/1
  Constant/1 -> Mux1/12
  PosGps/1 -> Mux1/11  "PosGPS"

== system pixhawk_slib_adv/CopterGroundModel/OnGroundFaceup ==
  Eular(rad) : Inport
  ModelInit_GroundSlope : Constant  Value=[0,0]
  Mux : Mux  Inputs=2
  Selector : Selector  InputPortWidth=3  IndexOptions=Index vector (dialog)  Indices=[3]  OutputSizes=1
  y : Outport
  wires:
  Mux/1 -> y/1
  ModelInit_GroundSlope/1 -> Mux/1
  Selector/1 -> Mux/2
  Eular(rad)/1 -> Selector/1

== system pixhawk_slib_adv/CopterMotorModel/MotorNonlinearDynamic1 ==
  Wb : Inport
  Cr : Inport  Port=2
  motorT : Inport  Port=3
  ModelInit_RPM : Inport  Port=4
  PWM : Inport  Port=5
  Minimum Throttle Cutoff : simulink/Logic and Bit Operations/Compare To Constant  relop=>=  const=ModelParam_motorMinThr  OutDataTypeStr=uint8
  Motor_Dynamics : Subsystem  TreatAsAtomicUnit=on
  Motor_Dynamics_backup : StateSpace  Commented=on  A=-1/ModelParam_motorT  C=1/ModelParam_motorT  D=0  InitialCondition=ModelInit_RPM*ModelParam_motorT
  Product : Product
  Product1 : Product
  Signal_Saturation : Saturate  UpperLimit=0.95  LowerLimit=0
  Sum1 : Sum  Inputs=++|
  radW : Outport
  wires:
  PWM/1 -> Signal_Saturation/1
  Motor_Dynamics/1(motor_rate_act) -> radW/1
  Product/1 -> Motor_Dynamics/1(motor_rate_d)
  Signal_Saturation/1 -> Product1/2, Minimum Throttle Cutoff/1
  Product1/1 -> Sum1/2
  Sum1/1 -> Product/1
  Wb/1 -> Sum1/1
  Minimum Throttle Cutoff/1 -> Product/2
  Cr/1 -> Product1/1
  motorT/1 -> Motor_Dynamics/3(motorT)
  ModelInit_RPM/1 -> Motor_Dynamics/2(ModelInit_RPM)

== system pixhawk_slib_adv/CopterMotorModel/MotorNonlinearDynamic2 ==
  Wb : Inport
  Cr : Inport  Port=2
  motorT : Inport  Port=3
  ModelInit_RPM : Inport  Port=4
  PWM : Inport  Port=5
  Minimum Throttle Cutoff : simulink/Logic and Bit Operations/Compare To Constant  relop=>=  const=ModelParam_motorMinThr  OutDataTypeStr=uint8
  Motor_Dynamics : Subsystem  TreatAsAtomicUnit=on
  Motor_Dynamics_backup : StateSpace  Commented=on  A=-1/ModelParam_motorT  C=1/ModelParam_motorT  D=0  InitialCondition=ModelInit_RPM*ModelParam_motorT
  Product : Product
  Product1 : Product
  Signal_Saturation : Saturate  UpperLimit=0.95  LowerLimit=0
  Sum1 : Sum  Inputs=++|
  radW : Outport
  wires:
  ModelInit_RPM/1 -> Motor_Dynamics/2(ModelInit_RPM)
  motorT/1 -> Motor_Dynamics/3(motorT)
  Cr/1 -> Product1/1
  Minimum Throttle Cutoff/1 -> Product/2
  Wb/1 -> Sum1/1
  Sum1/1 -> Product/1
  Product1/1 -> Sum1/2
  Signal_Saturation/1 -> Minimum Throttle Cutoff/1, Product1/2
  Product/1 -> Motor_Dynamics/1(motor_rate_d)
  Motor_Dynamics/1(motor_rate_act) -> radW/1
  PWM/1 -> Signal_Saturation/1

== system pixhawk_slib_adv/CopterMotorModel/MotorNonlinearDynamic3 ==
  Wb : Inport
  Cr : Inport  Port=2
  motorT : Inport  Port=3
  ModelInit_RPM : Inport  Port=4
  PWM : Inport  Port=5
  Minimum Throttle Cutoff : simulink/Logic and Bit Operations/Compare To Constant  relop=>=  const=ModelParam_motorMinThr  OutDataTypeStr=uint8
  Motor_Dynamics : Subsystem  TreatAsAtomicUnit=on
  Motor_Dynamics_backup : StateSpace  Commented=on  A=-1/ModelParam_motorT  C=1/ModelParam_motorT  D=0  InitialCondition=ModelInit_RPM*ModelParam_motorT
  Product : Product
  Product1 : Product
  Signal_Saturation : Saturate  UpperLimit=0.95  LowerLimit=0
  Sum1 : Sum  Inputs=++|
  radW : Outport
  wires:
  PWM/1 -> Signal_Saturation/1
  Motor_Dynamics/1(motor_rate_act) -> radW/1
  Product/1 -> Motor_Dynamics/1(motor_rate_d)
  Signal_Saturation/1 -> Product1/2, Minimum Throttle Cutoff/1
  Product1/1 -> Sum1/2
  Sum1/1 -> Product/1
  Wb/1 -> Sum1/1
  Minimum Throttle Cutoff/1 -> Product/2
  Cr/1 -> Product1/1
  motorT/1 -> Motor_Dynamics/3(motorT)
  ModelInit_RPM/1 -> Motor_Dynamics/2(ModelInit_RPM)

== system pixhawk_slib_adv/CopterMotorModel/MotorNonlinearDynamic4 ==
  Wb : Inport
  Cr : Inport  Port=2
  motorT : Inport  Port=3
  ModelInit_RPM : Inport  Port=4
  PWM : Inport  Port=5
  Minimum Throttle Cutoff : simulink/Logic and Bit Operations/Compare To Constant  relop=>=  const=ModelParam_motorMinThr  OutDataTypeStr=uint8
  Motor_Dynamics : Subsystem  TreatAsAtomicUnit=on
  Motor_Dynamics_backup : StateSpace  Commented=on  A=-1/ModelParam_motorT  C=1/ModelParam_motorT  D=0  InitialCondition=ModelInit_RPM*ModelParam_motorT
  Product : Product
  Product1 : Product
  Signal_Saturation : Saturate  UpperLimit=0.95  LowerLimit=0
  Sum1 : Sum  Inputs=++|
  radW : Outport
  wires:
  ModelInit_RPM/1 -> Motor_Dynamics/2(ModelInit_RPM)
  motorT/1 -> Motor_Dynamics/3(motorT)
  Cr/1 -> Product1/1
  Minimum Throttle Cutoff/1 -> Product/2
  Wb/1 -> Sum1/1
  Sum1/1 -> Product/1
  Product1/1 -> Sum1/2
  Signal_Saturation/1 -> Minimum Throttle Cutoff/1, Product1/2
  Product/1 -> Motor_Dynamics/1(motor_rate_d)
  Motor_Dynamics/1(motor_rate_act) -> radW/1
  PWM/1 -> Signal_Saturation/1

== system pixhawk_slib_adv/CopterMotorModel/MotorNonlinearDynamic5 ==
  Wb : Inport
  Cr : Inport  Port=2
  motorT : Inport  Port=3
  ModelInit_RPM : Inport  Port=4
  PWM : Inport  Port=5
  Minimum Throttle Cutoff : simulink/Logic and Bit Operations/Compare To Constant  relop=>=  const=ModelParam_motorMinThr  OutDataTypeStr=uint8
  Motor_Dynamics : Subsystem  TreatAsAtomicUnit=on
  Motor_Dynamics_backup : StateSpace  Commented=on  A=-1/ModelParam_motorT  C=1/ModelParam_motorT  D=0  InitialCondition=ModelInit_RPM*ModelParam_motorT
  Product : Product
  Product1 : Product
  Signal_Saturation : Saturate  UpperLimit=0.95  LowerLimit=0
  Sum1 : Sum  Inputs=++|
  radW : Outport
  wires:
  PWM/1 -> Signal_Saturation/1
  Motor_Dynamics/1(motor_rate_act) -> radW/1
  Product/1 -> Motor_Dynamics/1(motor_rate_d)
  Signal_Saturation/1 -> Product1/2, Minimum Throttle Cutoff/1
  Product1/1 -> Sum1/2
  Sum1/1 -> Product/1
  Wb/1 -> Sum1/1
  Minimum Throttle Cutoff/1 -> Product/2
  Cr/1 -> Product1/1
  motorT/1 -> Motor_Dynamics/3(motorT)
  ModelInit_RPM/1 -> Motor_Dynamics/2(ModelInit_RPM)

== system pixhawk_slib_adv/CopterMotorModel/MotorNonlinearDynamic6 ==
  Wb : Inport
  Cr : Inport  Port=2
  motorT : Inport  Port=3
  ModelInit_RPM : Inport  Port=4
  PWM : Inport  Port=5
  Minimum Throttle Cutoff : simulink/Logic and Bit Operations/Compare To Constant  relop=>=  const=ModelParam_motorMinThr  OutDataTypeStr=uint8
  Motor_Dynamics : Subsystem  TreatAsAtomicUnit=on
  Motor_Dynamics_backup : StateSpace  Commented=on  A=-1/ModelParam_motorT  C=1/ModelParam_motorT  D=0  InitialCondition=ModelInit_RPM*ModelParam_motorT
  Product : Product
  Product1 : Product
  Signal_Saturation : Saturate  UpperLimit=0.95  LowerLimit=0
  Sum1 : Sum  Inputs=++|
  radW : Outport
  wires:
  ModelInit_RPM/1 -> Motor_Dynamics/2(ModelInit_RPM)
  motorT/1 -> Motor_Dynamics/3(motorT)
  Cr/1 -> Product1/1
  Minimum Throttle Cutoff/1 -> Product/2
  Wb/1 -> Sum1/1
  Sum1/1 -> Product/1
  Product1/1 -> Sum1/2
  Signal_Saturation/1 -> Minimum Throttle Cutoff/1, Product1/2
  Product/1 -> Motor_Dynamics/1(motor_rate_d)
  Motor_Dynamics/1(motor_rate_act) -> radW/1
  PWM/1 -> Signal_Saturation/1

== system pixhawk_slib_adv/CopterMotorModel/MotorNonlinearDynamic7 ==
  Wb : Inport
  Cr : Inport  Port=2
  motorT : Inport  Port=3
  ModelInit_RPM : Inport  Port=4
  PWM : Inport  Port=5
  Minimum Throttle Cutoff : simulink/Logic and Bit Operations/Compare To Constant  relop=>=  const=ModelParam_motorMinThr  OutDataTypeStr=uint8
  Motor_Dynamics : Subsystem  TreatAsAtomicUnit=on
  Motor_Dynamics_backup : StateSpace  Commented=on  A=-1/ModelParam_motorT  C=1/ModelParam_motorT  D=0  InitialCondition=ModelInit_RPM*ModelParam_motorT
  Product : Product
  Product1 : Product
  Signal_Saturation : Saturate  UpperLimit=0.95  LowerLimit=0
  Sum1 : Sum  Inputs=++|
  radW : Outport
  wires:
  PWM/1 -> Signal_Saturation/1
  Motor_Dynamics/1(motor_rate_act) -> radW/1
  Product/1 -> Motor_Dynamics/1(motor_rate_d)
  Signal_Saturation/1 -> Product1/2, Minimum Throttle Cutoff/1
  Product1/1 -> Sum1/2
  Sum1/1 -> Product/1
  Wb/1 -> Sum1/1
  Minimum Throttle Cutoff/1 -> Product/2
  Cr/1 -> Product1/1
  motorT/1 -> Motor_Dynamics/3(motorT)
  ModelInit_RPM/1 -> Motor_Dynamics/2(ModelInit_RPM)

== system pixhawk_slib_adv/CopterMotorModel/MotorNonlinearDynamic8 ==
  Wb : Inport
  Cr : Inport  Port=2
  motorT : Inport  Port=3
  ModelInit_RPM : Inport  Port=4
  PWM : Inport  Port=5
  Minimum Throttle Cutoff : simulink/Logic and Bit Operations/Compare To Constant  relop=>=  const=ModelParam_motorMinThr  OutDataTypeStr=uint8
  Motor_Dynamics : Subsystem  TreatAsAtomicUnit=on
  Motor_Dynamics_backup : StateSpace  Commented=on  A=-1/ModelParam_motorT  C=1/ModelParam_motorT  D=0  InitialCondition=ModelInit_RPM*ModelParam_motorT
  Product : Product
  Product1 : Product
  Signal_Saturation : Saturate  UpperLimit=0.95  LowerLimit=0
  Sum1 : Sum  Inputs=++|
  radW : Outport
  wires:
  ModelInit_RPM/1 -> Motor_Dynamics/2(ModelInit_RPM)
  motorT/1 -> Motor_Dynamics/3(motorT)
  Cr/1 -> Product1/1
  Minimum Throttle Cutoff/1 -> Product/2
  Wb/1 -> Sum1/1
  Sum1/1 -> Product/1
  Product1/1 -> Sum1/2
  Signal_Saturation/1 -> Minimum Throttle Cutoff/1, Product1/2
  Product/1 -> Motor_Dynamics/1(motor_rate_d)
  Motor_Dynamics/1(motor_rate_act) -> radW/1
  PWM/1 -> Signal_Saturation/1

== system pixhawk_slib_adv/GroundModel/Subsystem1 ==
  In1 : Inport
  Bus Selector : BusSelector  OutputSignals=signal1,signal2
  PlaneGroundModel : pixhawk_slib_adv/PlaneGroundModel
      settings: SourceProductName=Pixhawk Target Blocks
  Out1 : Outport
  wires:
  Bus Selector/2 -> PlaneGroundModel/2  "<signal2>"
  Bus Selector/1 -> PlaneGroundModel/1  "<signal1>"
  PlaneGroundModel/1 -> Out1/1
  In1/1 -> Bus Selector/1

== system pixhawk_slib_adv/GroundModel/Subsystem2  ==
  In1 : Inport
  Bus Selector : BusSelector  OutputSignals=signal1,signal2
  CopterGroundModel : pixhawk_slib_adv/CopterGroundModel
      settings: SourceProductName=Pixhawk Target Blocks
  Out1 : Outport
  wires:
  Bus Selector/2 -> CopterGroundModel/2  "<signal2>"
  CopterGroundModel/1 -> Out1/1
  Bus Selector/1 -> CopterGroundModel/1  "<signal1>"
  In1/1 -> Bus Selector/1

== system pixhawk_slib_adv/PlaneGroundModel/OnGroundFaceup ==
  Eular(rad) : Inport
  ModelInit_GroundSlope : Constant  Value=[0,0]
  Mux : Mux  Inputs=2
  Selector : Selector  InputPortWidth=3  IndexOptions=Index vector (dialog)  Indices=[3]  OutputSizes=1
  y : Outport
  wires:
  Mux/1 -> y/1
  ModelInit_GroundSlope/1 -> Mux/1
  Selector/1 -> Mux/2
  Eular(rad)/1 -> Selector/1

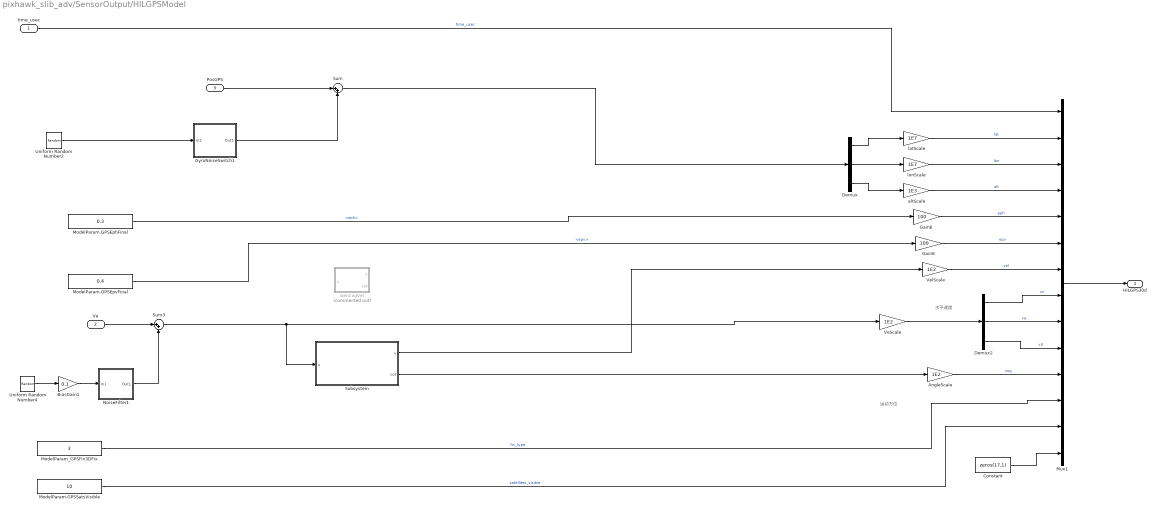
== system pixhawk_slib_adv/SensorOutput/HILGPSModel ==
  note: 水平速度
  note: 运动方位
  time_usec : Inport
  Ve : Inport  Port=2
  PosGPS : Inport  Port=3
  AngleScale : Gain  Gain=1E2
  BiasGain1 : Gain  Gain=0.1
  Constant : Constant  Value=zeros(17,1)
  Demux : Demux  Outputs=3
  Demux2 : Demux  Outputs=3
  Gain6 : Gain  Gain=100
  Gain8 : Gain  Gain=100
  GenCogVel : MATLAB Function  Commented=on  TreatAsAtomicUnit=on
  GyroNoiseSwitch1 : Subsystem
  ModelParam.GPSEphFinal : Constant  Value=0.3
  ModelParam.GPSEpvFinal : Constant  Value=0.4
  ModelParam.GPSSatsVisible : Constant  Value=10
  ModelParam_GPSFix3DFix : Constant  Value=3
  Mux1 : Mux  Inputs=14
  NoiseFilter1 : Subsystem
  Subsystem : Subsystem
  Sum : Sum  Inputs=|++
  Sum3 : Sum  Inputs=|++
  Uniform Random Number2 : UniformRandomNumber  Minimum=[-2.5e-6,-2.5e-6,-0.4]  Maximum=[2.5e-6,2.5e-6,0.4]  Seed=[1452,787,69]  SampleTime=0.001
  Uniform Random Number4 : UniformRandomNumber  Minimum=[-1,-1,-2]  Maximum=[1,1,2]  Seed=[5445,45433,33433]  SampleTime=0.001
  VeScale : Gain  Gain=1E2
  VelScale : Gain  Gain=1E2
  altScale : Gain  Gain=1E3
  latScale : Gain  Gain=1E7
  lonScale : Gain  Gain=1E7
  HILGPS30d : Outport
  wires:
  Gain6/1 -> Mux1/5  "eph"
  Gain8/1 -> Mux1/6  "epv"
  time_usec/1 -> Mux1/1  "time_usec"
  latScale/1 -> Mux1/2  "lat"
  lonScale/1 -> Mux1/3  "lon"
  altScale/1 -> Mux1/4  "alt"
  Demux2/1 -> Mux1/8  "vn"
  Demux2/2 -> Mux1/9  "ve"
  Demux2/3 -> Mux1/10  "vd"
  VeScale/1 -> Demux2/1
  VelScale/1 -> Mux1/7  "vel"
  AngleScale/1 -> Mux1/11  "cog"
  Sum/1 -> Demux/1
  Ve/1 -> Sum3/1
  Mux1/1 -> HILGPS30d/1
  BiasGain1/1 -> NoiseFilter1/1(In1)
  Uniform Random Number4/1 -> BiasGain1/1
  Sum3/1 -> Subsystem/1(u), VeScale/1
  NoiseFilter1/1(Out1) -> Sum3/2
  Demux/2 -> lonScale/1
  ModelParam.GPSEpvFinal/1 -> Gain8/1  "<epv>"
  Demux/3 -> altScale/1
  ModelParam.GPSEphFinal/1 -> Gain6/1  "<eph>"
  Subsystem/1(v) -> VelScale/1
  Subsystem/2(cot) -> AngleScale/1
  ModelParam.GPSSatsVisible/1 -> Mux1/13  "satellites_visible"
  ModelParam_GPSFix3DFix/1 -> Mux1/12  "fix_type"
  Demux/1 -> latScale/1
  Constant/1 -> Mux1/14
  Uniform Random Number2/1 -> GyroNoiseSwitch1/1(In1)
  PosGPS/1 -> Sum/1
  GyroNoiseSwitch1/1(Out1) -> Sum/2

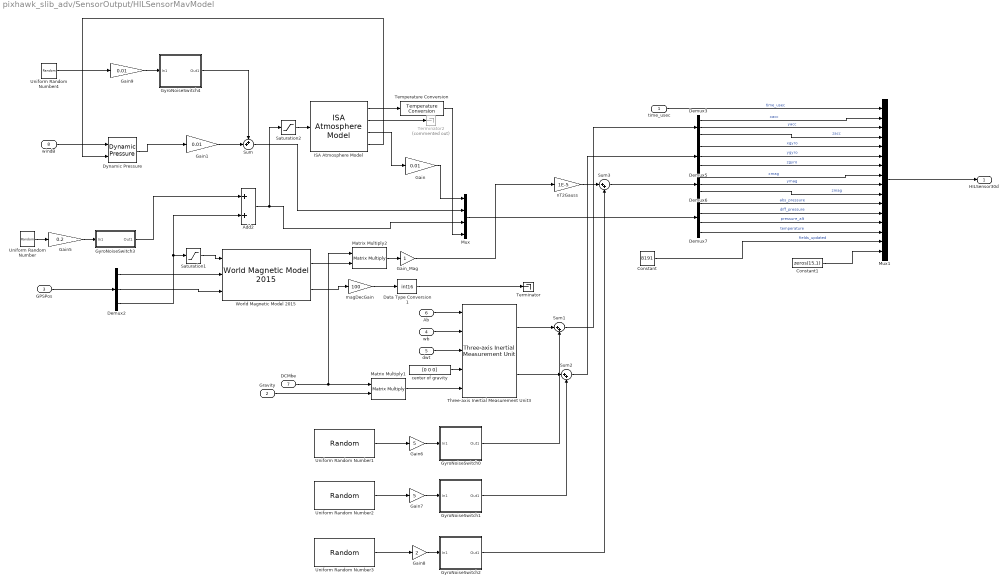
== system pixhawk_slib_adv/SensorOutput/HILSensorMavModel ==
  time_usec : Inport
  Gravity : Inport  Port=2
  GPSPos : Inport  Port=3
  wb : Inport  Port=4
  dwt : Inport  Port=5
  Ab : Inport  Port=6
  DCMbe : Inport  Port=7
  windB : Inport  Port=8
  Add2 : Sum
  Constant : Constant  Value=8191
  Constant1 : Constant  Value=zeros(15,1)
  Data Type Conversion1 : DataTypeConversion  OutDataTypeStr=int16
  Demux{2..3,5..6} (4 alike) : Demux  Outputs=3
  Demux7 : Demux
  Dynamic Pressure : aerolibasang/Dynamic Pressure
  Gain : Gain  Gain=0.01
  Gain1 : Gain  Gain=0.01
  Gain5 : Gain  Gain=0.2
  Gain6 : Gain  Gain=5
  Gain7 : Gain  Gain=5
  Gain8 : Gain  Gain=2
  Gain9 : Gain  Gain=0.01
  Gain_Mag : Gain
  GyroNoiseSwitch0 : Subsystem
  GyroNoiseSwitch1 : Subsystem
  GyroNoiseSwitch2 : Subsystem
  GyroNoiseSwitch3 : Subsystem
  GyroNoiseSwitch4 : Subsystem
  ISA Atmosphere Model : aerolibatmos2/ISA Atmosphere Model  custom=off  g=9.80665  gamma=1.4  R=287.0531  L=0.0065  h_trop=11000  h_strat=20000  rho0=1.225  P0=101325  T0=288.15  h0=0
      settings: SourceProductName=Aerospace Blockset
  Matrix Multiply1 : Product  Multiplication=Matrix(*)
  Matrix Multiply2 : Product  Multiplication=Matrix(*)
  Mux : Mux
  Mux1 : Mux  Inputs=16
  Saturation1 : Saturate  UpperLimit=100000  LowerLimit=0
  Saturation2 : Saturate  UpperLimit=100000  LowerLimit=0
  Sum : Sum  Inputs=++|
  Sum1 : Sum  Inputs=|++
  Sum2 : Sum  Inputs=|++
  Sum3 : Sum  Inputs=|++
  Temperature Conversion : aerolibconvert2/Temperature Conversion  IU=K  OU=C
      settings: SourceProductName=Aerospace Blockset  SourceProductBaseCode=AE
  Terminator : Terminator
  Terminator2 : Terminator  Commented=on
  Three-axis Inertial Measurement Unit3 : aerolibnav/Three-axis Inertial Measurement Unit  units=Metric (MKS)  imu=[0 0 0]  i_Ts=0  dtype_a=on  w_a=190  z_a=0.707  a_sf_cc=[1 0 0; 0 1 0; 0 0 1]  a_bias=[0 0 0]  a_sat="[-160  -160  -160 160 160 160]"  dtype_g=on  w_g=190  z_g=0.707  g_sf_cc=[1 0 0; 0 1 0; 0 0 1]  g_bias=[0 0 0]  g_sens=[0 0 0]  g_sat="[-4.36  -4.36  -4.36 4.36 4.36 4.36]"  i_rand=off  i_seeds=[23093 23094 23095 23096 23097 23098]  i_pow=ModelParam_noisePowerIMU*[0.0000005 0.0000005 0.0000005 0.000000002 0.000000002 0.000000002]
  Uniform Random Number : UniformRandomNumber  Minimum=-2  Maximum=2  Seed=15634  SampleTime=0.001
  Uniform Random Number1 : UniformRandomNumber  Minimum=-[0.1,0.1,0.2]  Maximum=[0.1,0.1,0.2]  Seed=[12233,645554,678766]  SampleTime=0.001
  Uniform Random Number2 : UniformRandomNumber  Minimum=-[0.01,0.01,0.01]  Maximum=[0.01,0.01,0.01]  Seed=[3243,44556,2334343]  SampleTime=0.001
  Uniform Random Number3 : UniformRandomNumber  Minimum=-[0.01,0.01,0.01]  Maximum=[0.01,0.01,0.01]  Seed=[45465,454534,1234232]  SampleTime=0.001
  Uniform Random Number4 : UniformRandomNumber  Seed=25634  SampleTime=0.001
  World Magnetic Model 2015 : aerolibgravity2/World Magnetic Model 2015  units=Metric (MKS)  time_in=off  month=November  day=3  year=2017  action=Error  h_out=off  dec_out=on  inc_out=off  ti_out=off
      settings: SourceProductName=Aerospace Blockset  SourceProductBaseCode=AE
  center of gravity : Constant  Value=[0 0 0]
  magDecGain : Gain  Gain=100
  nT2Gauss : Gain  Gain=1E-5
  HILSensor30d : Outport
  wires:
  center of gravity/1 -> Three-axis Inertial Measurement Unit3/4
  Matrix Multiply2/1 -> Gain_Mag/1
  magDecGain/1 -> Data Type Conversion1/1
  GyroNoiseSwitch3/1(Out1) -> Add2/1
  ISA Atmosphere Model/4 -> Dynamic Pressure/2
  windB/1 -> Dynamic Pressure/1
  Uniform Random Number/1 -> Gain5/1
  dwt/1 -> Three-axis Inertial Measurement Unit3/3
  Gain_Mag/1 -> nT2Gauss/1
  Dynamic Pressure/1 -> Gain1/1
  Add2/1 -> Mux/3, Saturation2/1
  Demux2/3 -> Saturation1/1, Add2/2
  Demux2/2 -> World Magnetic Model 2015/3
  Demux2/1 -> World Magnetic Model 2015/2
  Matrix Multiply1/1 -> Three-axis Inertial Measurement Unit3/5
  DCMbe/1 -> Matrix Multiply2/1, Matrix Multiply1/1
  Gravity/1 -> Matrix Multiply1/2
  Sum/1 -> Mux/2
  Gain/1 -> Mux/1
  Constant/1 -> Mux1/15  "fields_updated"
  time_usec/1 -> Mux1/1  "time_usec"
  Demux7/2 -> Mux1/12  "diff_pressure"
  Demux7/3 -> Mux1/13  "pressure_alt"
  Demux6/2 -> Mux1/9  "ymag"
  Demux6/3 -> Mux1/10  "zmag"
  Demux7/1 -> Mux1/11  "abs_pressure"
  Demux5/2 -> Mux1/6  "ygyro"
  Demux6/1 -> Mux1/8  "xmag"
  Demux5/3 -> Mux1/7  "zgyro"
  Demux7/4 -> Mux1/14  "temperature"
  Demux3/1 -> Mux1/2  "xacc"
  Demux3/2 -> Mux1/3  "yacc"
  Demux5/1 -> Mux1/5  "xgyro"
  Demux3/3 -> Mux1/4  "zacc"
  Ab/1 -> Three-axis Inertial Measurement Unit3/1
  wb/1 -> Three-axis Inertial Measurement Unit3/2
  nT2Gauss/1 -> Sum3/1
  Gain8/1 -> GyroNoiseSwitch2/1(In1)
  GyroNoiseSwitch1/1(Out1) -> Sum2/2
  GyroNoiseSwitch2/1(Out1) -> Sum3/2
  Sum1/1 -> Demux3/1
  Sum2/1 -> Demux5/1
  Sum3/1 -> Demux6/1
  Mux/1 -> Demux7/1
  Mux1/1 -> HILSensor30d/1
  Data Type Conversion1/1 -> Terminator/1
  Three-axis Inertial Measurement Unit3/1 -> Sum1/1
  Three-axis Inertial Measurement Unit3/2 -> Sum2/1
  ISA Atmosphere Model/2 -> Terminator2/1
  Gain5/1 -> GyroNoiseSwitch3/1(In1)
  GyroNoiseSwitch0/1(Out1) -> Sum1/2
  Uniform Random Number1/1 -> Gain6/1
  Gain7/1 -> GyroNoiseSwitch1/1(In1)
  Uniform Random Number2/1 -> Gain7/1
  Uniform Random Number3/1 -> Gain8/1
  ISA Atmosphere Model/3 -> Gain/1
  Gain6/1 -> GyroNoiseSwitch0/1(In1)
  Gain9/1 -> GyroNoiseSwitch4/1(In1)
  Uniform Random Number4/1 -> Gain9/1
  Gain1/1 -> Sum/2
  GyroNoiseSwitch4/1(Out1) -> Sum/1
  Saturation1/1 -> World Magnetic Model 2015/1
  Saturation2/1 -> ISA Atmosphere Model/1
  World Magnetic Model 2015/2 -> magDecGain/1
  World Magnetic Model 2015/1 -> Matrix Multiply2/2
  GPSPos/1 -> Demux2/1
  Constant1/1 -> Mux1/16
  ISA Atmosphere Model/1 -> Temperature Conversion/1
  Temperature Conversion/1 -> Mux/4

== system pixhawk_slib_adv/sendUE4ExtAct/Ue4ExtMsgEncoder ==
  note: struct Ue4ExtMsg {
      | int checksum ;
      | int CopterID ;
      | double runnedTime ; //Current stamp (s)
      | float pwm [ 16 ];
      | }
      |
      | This struct should be sent to 20010 port
      | The checksum should be 1234567894
      | This msg defines the 9-24 actuators of CopterID
  copterID : Inport  PortDimensions=1
  pwm : Inport  Port=2  PortDimensions=16
  Data Type Conversion : DataTypeConversion  OutDataTypeStr=int32
  Data Type Conversion1 : DataTypeConversion  OutDataTypeStr=single
  Data Type Conversion2 : DataTypeConversion  OutDataTypeStr=double
  Mux1 : Mux  Inputs=2
  PayLoad : etargetslib/Byte Pack  datatypes={'int32','double','single'}  byteAlign=4
  checkSum : Constant  Value=1234567894
  runnedTime1 : Clock
  Ue4ExtMsg : Outport
  wires:
  copterID/1 -> Mux1/2
  pwm/1 -> Data Type Conversion1/1
  runnedTime1/1 -> Data Type Conversion2/1
  Mux1/1 -> Data Type Conversion/1
  PayLoad/1 -> Ue4ExtMsg/1
  checkSum/1 -> Mux1/1
  Data Type Conversion1/1 -> PayLoad/3
  Data Type Conversion2/1 -> PayLoad/2
  Data Type Conversion/1 -> PayLoad/1

== system pixhawk_slib_adv/sendUE4Pos2Ground/Subsystem10 ==
  copterID : Inport  PortDimensions=1
  vehicleType : Inport  Port=2  PortDimensions=1
  PosE : Inport  Port=3  PortDimensions=3
  AngEuler : Inport  Port=4  PortDimensions=3
  Clock : Clock
  Constant{,3..5} (4 alike) : Constant  Value=[0,0,0]
  Constant1 : Constant  Value=[0,0,0,0]
  Constant2 : Constant  Value=ones(8,1)*3000
  Subsystem : Subsystem
  toUnReal : Outport
  wires:
  Constant/1 -> Subsystem/4("VelE ")
  PosE/1 -> Subsystem/5(PosE)
  vehicleType/1 -> Subsystem/2(vehicleType)
  Clock/1 -> Subsystem/3(runnedTime)
  Constant4/1 -> Subsystem/10(RateB)
  Constant5/1 -> Subsystem/11(PosGPS)
  AngEuler/1 -> Subsystem/6(AngEuler)
  Subsystem/1(toUnReal) -> toUnReal/1
  Constant3/1 -> Subsystem/9(AccB)
  Constant1/1 -> Subsystem/7(AngQuatern)
  copterID/1 -> Subsystem/1(copterID)
  Constant2/1 -> Subsystem/8(MotorRPMS)

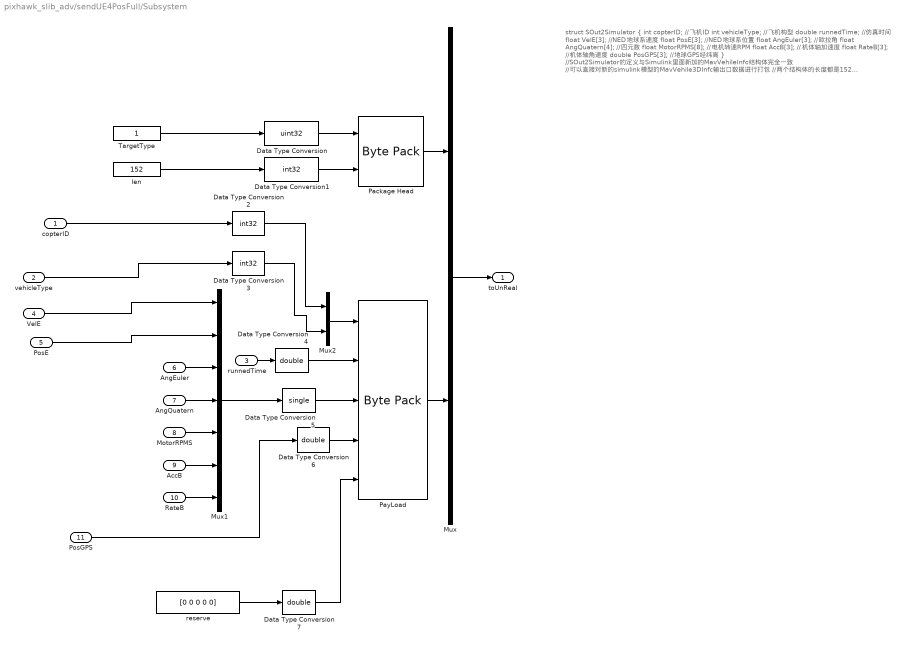
== system pixhawk_slib_adv/sendUE4PosFull/Subsystem ==
  note: struct SOut2Simulator
      | {
      | int copterID; //飞机ID
      | int vehicleType; //飞机构型
      | double runnedTime; //仿真时间
      | float VelE[3]; //NED地球系速度
      | float PosE[3]; //NED地球系位置
      | float AngEuler[3]; //欧拉角
      | float AngQuatern[4]; //四元数
      | float MotorRPMS[8]; //电机转速RPM
      | float AccB[3]; //机体轴加速度
      | float RateB[3]; //机体轴角速度
      | double PosGPS[3]; //地球GPS经纬高
      | }
      |
      | //SOut2Simulator的定义与Simulink里面新加的MavVehileInfo结构体完全一致
      | //可以直接对新的simulink模型的MavVehile3DInfo输出口数据进行打包
      | //两个结构体的长度都是152
      | sizeof(SOut2Simulator) = sizeof(MavVehileInfo) = 152
      |
      | 打包封装的结构体为
      | typedef struct _netDataShort
      | {
      | TargetType tg; //这里目前随便填，写1即可 uint32
      | int len; //这个长度为传输结构体长度，目前是152
      | char payload[192]; //这里面前152位存放了SOut2Simulator结构体数据，后面的40位保留
      | }netDataShort;
      |
      | //UDP包的总长度为200
      | sizeof(netDataShort) = 200
      |
      | //发送的UDP端口号为：20010
  copterID : Inport  PortDimensions=1
  vehicleType : Inport  Port=2  PortDimensions=1
  runnedTime : Inport  Port=3  PortDimensions=1
  "VelE " : Inport  Port=4  PortDimensions=3
  PosE : Inport  Port=5  PortDimensions=3
  AngEuler : Inport  Port=6  PortDimensions=3
  AngQuatern : Inport  Port=7  PortDimensions=4
  MotorRPMS : Inport  Port=8
  AccB : Inport  Port=9  PortDimensions=3
  RateB : Inport  Port=10  PortDimensions=3
  PosGPS : Inport  Port=11  PortDimensions=3
  Data Type Conversion : DataTypeConversion  OutDataTypeStr=uint32
  Data Type Conversion1 : DataTypeConversion  OutDataTypeStr=int32
  Data Type Conversion2 : DataTypeConversion  OutDataTypeStr=int32
  Data Type Conversion3 : DataTypeConversion  OutDataTypeStr=int32
  Data Type Conversion4 : DataTypeConversion  OutDataTypeStr=double
  Data Type Conversion5 : DataTypeConversion  OutDataTypeStr=single
  Data Type Conversion6 : DataTypeConversion  OutDataTypeStr=double
  Data Type Conversion7 : DataTypeConversion  OutDataTypeStr=double
  Mux : Mux  Inputs=2
  Mux1 : Mux  Inputs=7
  Mux2 : Mux  Inputs=2
  Package Head : etargetslib/Byte Pack  datatypes={'uint32','int32'}  byteAlign=4
  PayLoad : etargetslib/Byte Pack  datatypes={'int32','double','single','double','double'}  byteAlign=8
  TargetType : Constant  OutDataTypeStr=Inherit: Inherit via back propagation
  len : Constant  Value=152  OutDataTypeStr=Inherit: Inherit via back propagation
  reserve : Constant  Value=[0 0 0 0 0]  OutDataTypeStr=double
  toUnReal : Outport
  wires:
  runnedTime/1 -> Data Type Conversion4/1
  RateB/1 -> Mux1/7
  PayLoad/1 -> Mux/2
  "VelE "/1 -> Mux1/1
  Mux1/1 -> Data Type Conversion5/1
  PosGPS/1 -> Data Type Conversion6/1
  Package Head/1 -> Mux/1
  AccB/1 -> Mux1/6
  Mux/1 -> toUnReal/1
  MotorRPMS/1 -> Mux1/5
  AngQuatern/1 -> Mux1/4
  copterID/1 -> Data Type Conversion2/1
  len/1 -> Data Type Conversion1/1
  vehicleType/1 -> Data Type Conversion3/1
  PosE/1 -> Mux1/2
  TargetType/1 -> Data Type Conversion/1
  reserve/1 -> Data Type Conversion7/1
  Mux2/1 -> PayLoad/1
  AngEuler/1 -> Mux1/3
  Data Type Conversion5/1 -> PayLoad/3
  Data Type Conversion2/1 -> Mux2/1
  Data Type Conversion1/1 -> Package Head/2
  Data Type Conversion6/1 -> PayLoad/4
  Data Type Conversion/1 -> Package Head/1
  Data Type Conversion3/1 -> Mux2/2
  Data Type Conversion4/1 -> PayLoad/2
  Data Type Conversion7/1 -> PayLoad/5
